simulink model "VSMr_2023b"  (R2023b)
settings: Solver=ode14x  StartTime=0  StopTime=Sim.tend  FixedStep=0.000125  RelTol=4e-4
model workspace (MAT data in the model file):
  nr_vsm : Simulink.Parameter (value not decoded)
values from neighbouring files (symbols this model uses):
  ControlSampleTime = 1/8000    (= 0.000125)    [sim3run_390.m]
  ddfmax = 60    [prm3var_390.m]
  T_seccontrol = 20    [prm3var_390.m]
  Ts = TS    [sim3run_390.m]
  TVRint = 0.85    [prm3var_390.m]
  vsm_Tdaco = 0.01    [prm3var_390.m]
symbols that are objects in the model workspace (value not decoded): nr_vsm
undefined symbols (not defined in the file or in its folder): DiscIntNeverNeededParam, General, parameterset, prm_vsm, pu_vsm, UFLS, VSM
libraries: simulink x55, FriedrichLibrary x10, simulink_extras x2, spsSampleandHoldLib x2
(part 2 of 3)

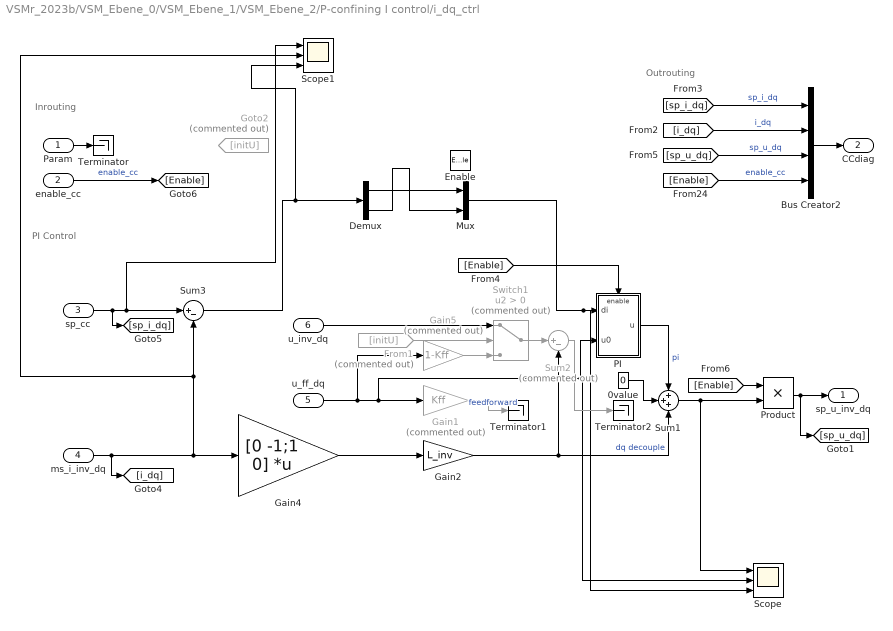
== system VSMr_2023b/VSM_Ebene_0/VSM_Ebene_1/VSM_Ebene_2/P-confining I control/i_dq_ctrl ==
  note: Inrouting
  note: Outrouting
  note: PI Control
  Param : Inport
  enable_cc : Inport  Port=2
  sp_cc : Inport  Port=3
  ms_i_inv_dq : Inport  Port=4
  u_ff_dq : Inport  Port=5
  u_inv_dq : Inport  Port=6
  Enable : EnablePort  StatesWhenEnabling=reset
  0value : Constant  Value=0
  Bus Creator2 : BusCreator  Inputs=4
  Demux : Demux  Outputs=2
  From1 : From  Commented=on  GotoTag=initU
  Gain1 : Gain  Commented=on  Gain=Kff
  Gain2 : Gain  Gain=L_inv
  Gain4 : Gain  Gain=[0 -1;1 0]  Multiplication=Matrix(K*u)
  Gain5 : Gain  Commented=on  Gain=1-Kff
  Goto2 : Goto  Commented=on  GotoTag=initU
  Mux : Mux  Inputs=2
  PI : Subsystem
  Product : Product
  Scope : Scope  NumInputPorts=3
  Scope1 : Scope  NumInputPorts=3
  Sum1 : Sum  Inputs=+++
  Sum2 : Sum  Commented=on  Inputs=|+-
  Sum3 : Sum  Inputs=|+-
  Switch1 : Switch  Commented=on  Criteria=u2 > Threshold  SaturateOnIntegerOverflow=off  InputSameDT=off
  Terminator : Terminator
  Terminator1 : Terminator
  Terminator2 : Terminator
  sp_u_inv_dq : Outport  VectorParamsAs1DForOutWhenUnconnected=off
  CCdiag : Outport  Port=2  VectorParamsAs1DForOutWhenUnconnected=off
  wires:
  Switch1/1 -> Sum2/1
  Gain4/1 -> Gain2/1
  Gain2/1 -> Sum1/3, Sum2/2  "dq decouple"
  From1/1 -> Switch1/2
  Sum1/1 -> Scope/1, Product/2
  u_inv_dq/1 -> Switch1/1
  [Enable] -> PI/Enable
  Sum3/1 -> Demux/1, Scope1/3
  sp_cc/1 -> [sp_i_dq], Scope1/1, Sum3/1
  Param/1 -> Terminator/1
  [Enable] -> Product/1
  [sp_u_dq] -> Bus Creator2/3  "sp_u_dq"
  enable_cc/1 -> [Enable]  "enable_cc"
  [Enable] -> Bus Creator2/4  "enable_cc"
  Bus Creator2/1 -> CCdiag/1
  [sp_i_dq] -> Bus Creator2/1  "sp_i_dq"
  [i_dq] -> Bus Creator2/2  "i_dq"
  u_ff_dq/1 -> PI/2(u0), Scope/2, Gain1/1, Gain5/1
  Gain5/1 -> Switch1/3
  Product/1 -> sp_u_inv_dq/1, [sp_u_dq]
  ms_i_inv_dq/1 -> [i_dq], Scope1/2, Sum3/2, Gain4/1
  Mux/1 -> Scope/3, PI/1(di)
  Demux/2 -> Mux/2
  Demux/1 -> Mux/1
  PI/1(u) -> Sum1/1  "pi"
  Gain1/1 -> Terminator1/1  "feedforward"
  Sum2/1 -> Terminator2/1
  0value/1 -> Sum1/2

== system VSMr_2023b/VSM_Ebene_0/VSM_Ebene_1/VSM_Ebene_2/VSM_Ebene_3/Angle Integrator [SI] ==
  omega : Inport
  phi0 : Inport  Port=2
  Bias : Bias  Bias=-2*pi  SaturateOnIntegerOverflow=off
  Bias1 : Bias  Bias=2*pi  SaturateOnIntegerOverflow=off
  Delay : Delay  DelayLength=1  InitialConditionSource=Input port  SampleTime=Ts
      settings: InputPortMap=u0,p4
  Delay1 : Delay  DelayLength=1  InitialConditionSource=Input port  SampleTime=Ts
      settings: InputPortMap=u0,p4
  Gain3 : Gain  Gain=Ts
  Sum : Sum  Inputs=|++
  Sum1 : Sum  Inputs=|++
  Switch : Switch  Criteria=u2 > Threshold  Threshold=pi  SaturateOnIntegerOverflow=off  InputSameDT=off
  Switch1 : Switch  Threshold=-pi  SaturateOnIntegerOverflow=off  InputSameDT=off
  phi : Outport  VectorParamsAs1DForOutWhenUnconnected=off
  phi_acc : Outport  Port=2  VectorParamsAs1DForOutWhenUnconnected=off
  wires:
  Delay1/1 -> Sum1/2, phi_acc/1
  Sum1/1 -> Delay1/1
  Gain3/1 -> Sum/1, Sum1/1
  phi0/1 -> Delay/2, Delay1/2
  omega/1 -> Gain3/1
  Bias/1 -> Switch/1
  Sum/1 -> Switch/3, Switch/2, Bias/1
  Delay/1 -> Sum/2, phi/1
  Switch/1 -> Switch1/1, Bias1/1, Switch1/2
  Bias1/1 -> Switch1/3
  Switch1/1 -> Delay/1

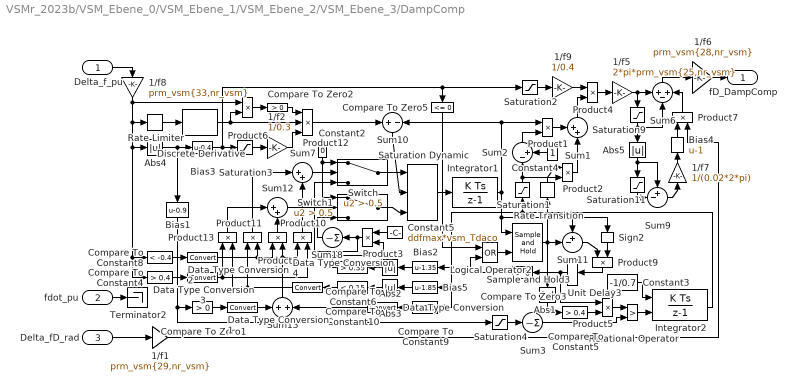
== system VSMr_2023b/VSM_Ebene_0/VSM_Ebene_1/VSM_Ebene_2/VSM_Ebene_3/DampComp ==
  Delta_f_pu : Inport
  fdot_pu : Inport  Port=2
  Delta_fD_rad : Inport  Port=3
  1/f1 : Gain  Gain=prm_vsm{29,nr_vsm}
  1/f2 : Gain  Gain=1/0.3
  1/f5 : Gain  Gain=2*pi*prm_vsm{25,nr_vsm}
  1/f6 : Gain  Gain=prm_vsm{28,nr_vsm}
  1/f7 : Gain  Gain=1/(0.02*2*pi)
  1/f8 : Gain  Gain=prm_vsm{33,nr_vsm}
  1/f9 : Gain  Gain=1/0.4
  Abs{1..5} (5 alike) : Abs  SaturateOnIntegerOverflow=off
  Bias1 : Bias  Bias=-0.9  SaturateOnIntegerOverflow=off
  Bias2 : Bias  Bias=-1.35  SaturateOnIntegerOverflow=off
  Bias3 : Bias  Bias=-0.4  SaturateOnIntegerOverflow=off
  Bias4 : Bias  Bias=-1  SaturateOnIntegerOverflow=off
  Bias5 : Bias  Bias=-1.85  SaturateOnIntegerOverflow=off
  Compare To Constant10 : simulink/Logic and Bit Operations/Compare To Constant  relop=<  const=0.15  OutDataTypeStr=boolean
  Compare To Constant4 : simulink/Logic and Bit Operations/Compare To Constant  relop=>  const=0.4  OutDataTypeStr=boolean
  Compare To Constant5 : simulink/Logic and Bit Operations/Compare To Constant  relop=>  const=0.4  OutDataTypeStr=boolean
  Compare To Constant6 : simulink/Logic and Bit Operations/Compare To Constant  relop=>  const=0.35  OutDataTypeStr=boolean
  Compare To Constant8 : simulink/Logic and Bit Operations/Compare To Constant  relop=<  const=-0.4  OutDataTypeStr=boolean
  Compare To Constant9 : simulink/Logic and Bit Operations/Compare To Constant  relop=<  const=1.5  OutDataTypeStr=boolean
  Compare To Zero1 : simulink/Logic and Bit Operations/Compare To Zero  relop=>  OutDataTypeStr=boolean
  Compare To Zero2 : simulink/Logic and Bit Operations/Compare To Zero  relop=>  OutDataTypeStr=boolean
  Compare To Zero3 : simulink/Logic and Bit Operations/Compare To Zero  relop=>  OutDataTypeStr=boolean
  Compare To Zero5 : simulink/Logic and Bit Operations/Compare To Zero  relop=<=  OutDataTypeStr=boolean
  Constant2 : Constant  Value=0
  Constant3 : Constant  Value=-1/0.7
  Constant4 : Constant
  Constant5 : Constant  Value=ddfmax*vsm_Tdaco
  Data Type Conversion{,1..4} (5 alike) : DataTypeConversion  SaturateOnIntegerOverflow=off  RndMeth=Floor
  Discrete Derivative : simulink/Discrete/Discrete Derivative  gainval=1.0  ICPrevScaledInput=0.0  OutMin=[]  OutMax=[]  OutDataType=fixdt(1, 16)  OutScaling=2^-10  DoSatur=off
  Integrator1 : DiscreteIntegrator  gainval=1/vsm_Tdaco  SampleTime=-1  LimitOutput=on  UpperSaturationLimit=4  LowerSaturationLimit=-4  ICPrevOutput=DiscIntNeverNeededParam  ICPrevScaledInput=DiscIntNeverNeededParam
  Integrator2 : DiscreteIntegrator  gainval=1  ExternalReset=level  InitialCondition=2.001  SampleTime=-1  LimitOutput=on  UpperSaturationLimit=2.001  LowerSaturationLimit=0  ICPrevOutput=DiscIntNeverNeededParam  ICPrevScaledInput=DiscIntNeverNeededParam
  Logical Operator2 : Logic  Operator=OR  AllPortsSameDT=off  OutDataTypeStr=boolean
  Product{1..11,13} (12 alike) : Product
  Product12 : Product  Inputs=3
  Rate Limiter : RateLimiter  RisingSlewLimit=4  FallingSlewLimit=-4  SampleTimeMode=inherited
  Rate Transition : RateTransition  Integrity=off  InitialCondition=-1  OutPortSampleTime=ControlSampleTime
  Relational Operator : RelationalOperator  Operator=>  OutDataTypeStr=boolean  RndMeth=Simplest  InputSameDT=off
  Sample and Hold3 : spsSampleandHoldLib/Sample and Hold  ic=0  Ts=0
  Saturation Dynamic : simulink/Discontinuities/Saturation Dynamic  OutMin=[]  OutMax=[]  OutDataTypeStr=Inherit: Same as second input  OutDataType=fixdt(1, 16)  OutScaling=2^-10  DoSatur=off
  Saturation1 : Saturate  UpperLimit=1  LowerLimit=0
  Saturation11 : Saturate  UpperLimit=0.02*2*pi  LowerLimit=0
  Saturation2 : Saturate  UpperLimit=0.4  LowerLimit=0
  Saturation3 : Saturate  UpperLimit=0.3  LowerLimit=0
  Saturation4 : Saturate  UpperLimit=0.3  LowerLimit=0.01
  Saturation9 : Saturate  UpperLimit=0.04*2*pi  LowerLimit=-0.04*2*pi
  Sign2 : Signum
  Sum1 : Sum  Inputs=++|
  Sum10 : Sum  Inputs=+|-
  Sum11 : Sum  Inputs=+-|
  Sum12 : Sum  Inputs=|++
  Sum13 : Sum  Inputs=+|+
  Sum18 : Sum  Inputs=|-|
  Sum2 : Sum  Inputs=|-+
  Sum3 : Sum  Inputs=-
  Sum6 : Sum  Inputs=+-+
  Sum7 : Sum  Inputs=|++
  Sum9 : Sum  Inputs=+-|
  Switch : Switch  Criteria=u2 > Threshold  Threshold=0.5  SaturateOnIntegerOverflow=off  InputSameDT=off
  Switch1 : Switch  Criteria=u2 > Threshold  Threshold=0.5  SaturateOnIntegerOverflow=off  InputSameDT=off
  Terminator2 : Terminator
  Unit Delay3 : UnitDelay  SampleTime=-1  HasFrameUpgradeWarning=on
  fD_DampComp : Outport
  wires:
  fdot_pu/1 -> Terminator2/1
  Delta_f_pu/1 -> 1/f8/1
  Delta_fD_rad/1 -> 1/f1/1
  Product7/1 -> Sum6/3
  Saturation9/1 -> Sum6/2, Abs5/1
  1/f7/1 -> Bias4/1
  Abs5/1 -> Sum9/1, Saturation11/1
  Saturation11/1 -> Sum9/2
  Sum9/1 -> 1/f7/1
  Bias4/1 -> Product7/1
  1/f5/1 -> Sum6/1, Saturation9/1
  1/f8/1 -> Abs4/1, Compare To Constant4/1, Compare To Constant8/1, Rate Limiter/1, Product6/1
  Sum10/1 -> Saturation Dynamic/2
  Product12/1 -> Sum10/1
  Saturation Dynamic/1 -> Integrator1/1
  Bias3/1 -> Saturation2/1, Compare To Zero5/1, Saturation3/1
  Integrator1/1 -> Product1/1, Sum10/2, Sample and Hold3/1, Sign2/1, Sum11/1
  Sum11/1 -> Product9/1
  Product5/1 -> Relational Operator/1
  Switch/1 -> Saturation Dynamic/1
  Constant2/1 -> Switch1/1, Switch/1
  Switch1/1 -> Saturation Dynamic/3
  Product3/1 -> Switch/3, Sum18/1
  Sum18/1 -> Switch1/3
  Sum6/1 -> 1/f6/1
  1/f1/1 -> Product7/2
  Compare To Zero5/1 -> Logical Operator2/1
  Product4/1 -> 1/f5/1
  Product2/1 -> Sum1/2
  Product1/1 -> Sum1/1
  Saturation1/1 -> Sum2/1, Product2/2
  Compare To Zero3/1 -> Logical Operator2/2
  Sum2/1 -> Product1/2
  Sample and Hold3/1 -> Rate Transition/1, Abs1/1, Sum11/2
  Constant5/1 -> Product3/1
  1/f6/1 -> fD_DampComp/1
  Sum1/1 -> Product4/2
  1/f9/1 -> Product4/1
  Saturation2/1 -> 1/f9/1
  1/f2/1 -> Product12/3
  Abs1/1 -> Compare To Constant5/1
  Compare To Constant5/1 -> Product5/2
  Product6/1 -> Compare To Zero2/1
  Compare To Zero2/1 -> Product12/1
  Bias2/1 -> Abs2/1
  Abs2/1 -> Compare To Constant6/1
  Compare To Constant6/1 -> Product3/2
  Sum7/1 -> Switch/2
  Compare To Constant4/1 -> Data Type Conversion3/1
  Sum12/1 -> Switch1/2
  Compare To Constant8/1 -> Data Type Conversion2/1
  Unit Delay3/1 -> Compare To Zero3/1, Product5/1
  Relational Operator/1 -> Integrator2/2
  Integrator2/1 -> Bias2/1, Bias5/1, Compare To Constant9/1, Saturation1/1
  Compare To Constant9/1 -> Data Type Conversion/1
  Bias5/1 -> Abs3/1
  Abs3/1 -> Compare To Constant10/1
  Product8/1 -> Sum12/2
  Sum13/1 -> Product8/2, Product10/1
  Abs4/1 -> Bias1/1, Bias3/1
  Product10/1 -> Sum7/2
  Product13/1 -> Sum12/1
  Compare To Constant10/1 -> Data Type Conversion4/1
  Product11/1 -> Sum7/1
  Data Type Conversion/1 -> Sum13/2
  Data Type Conversion1/1 -> Sum13/1
  Data Type Conversion2/1 -> Product11/2, Product8/1
  Data Type Conversion3/1 -> Product13/1, Product10/2
  Data Type Conversion4/1 -> Product11/1, Product13/2
  Discrete Derivative/1 -> Product12/2, Product6/2
  Rate Limiter/1 -> Discrete Derivative/1
  Sign2/1 -> Product9/2
  Saturation3/1 -> 1/f2/1
  Compare To Zero1/1 -> Data Type Conversion1/1
  Bias1/1 -> Saturation4/1, Compare To Zero1/1
  Sum3/1 -> Relational Operator/2
  Saturation4/1 -> Sum3/1
  Rate Transition/1 -> Product2/1
  Constant3/1 -> Integrator2/1
  Constant4/1 -> Sum2/2
  Product9/1 -> Unit Delay3/1
  Logical Operator2/1 -> Sample and Hold3/2

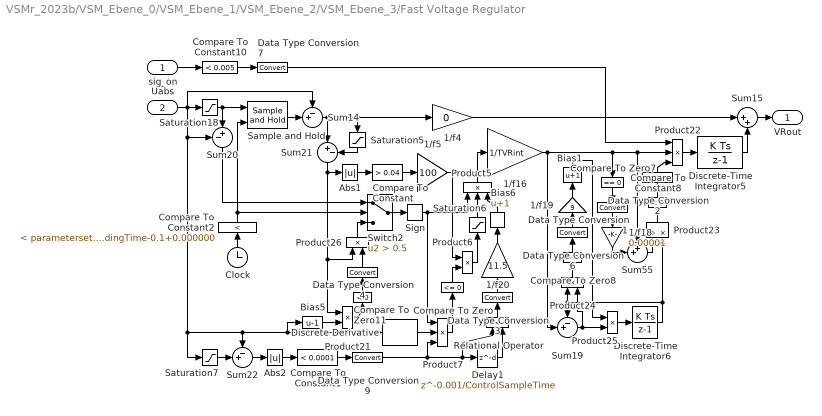
== system VSMr_2023b/VSM_Ebene_0/VSM_Ebene_1/VSM_Ebene_2/VSM_Ebene_3/Fast Voltage Regulator ==
  sig_on : Inport
  Uabs : Inport  Port=2  SampleTime=ControlSampleTime
  1/f16 : Gain  Gain=1/TVRint
  1/f18 : Gain  Gain=0.00001
  1/f19 : Gain  Gain=9
  1/f20 : Gain  Gain=11.5
  1/f4 : Gain  Gain=0
  1/f5 : Gain  Gain=100
  Abs1 : Abs  SaturateOnIntegerOverflow=off
  Abs2 : Abs  SaturateOnIntegerOverflow=off
  Bias1 : Bias  Bias=1  SaturateOnIntegerOverflow=off
  Bias5 : Bias  Bias=-1  SaturateOnIntegerOverflow=off
  Bias6 : Bias  Bias=1  SaturateOnIntegerOverflow=off
  Clock : Clock
  Compare To Constant : simulink/Logic and Bit Operations/Compare To Constant  relop=>  const=0.04  OutDataTypeStr=boolean
  Compare To Constant1 : simulink/Logic and Bit Operations/Compare To Constant  relop=<  const=0.0001  OutDataTypeStr=boolean
  Compare To Constant10 : simulink/Logic and Bit Operations/Compare To Constant  relop=<  const=0.005  OutDataTypeStr=boolean
  Compare To Constant2 : simulink/Logic and Bit Operations/Compare To Constant  relop=<  const=parameterset.Event.IslandingTime-0.1+0.000000  OutDataTypeStr=boolean
  Compare To Constant8 : simulink/Logic and Bit Operations/Compare To Constant  relop=<  const=2  OutDataTypeStr=boolean
  Compare To Zero : simulink/Logic and Bit Operations/Compare To Zero  relop=<=  OutDataTypeStr=boolean
  Compare To Zero11 : simulink/Logic and Bit Operations/Compare To Zero  relop=<  OutDataTypeStr=boolean
  Compare To Zero7 : simulink/Logic and Bit Operations/Compare To Zero  relop===  OutDataTypeStr=boolean
  Compare To Zero8 : simulink/Logic and Bit Operations/Compare To Zero  relop=>  OutDataTypeStr=boolean
  Data Type Conversion{1..4,6..7,9} (7 alike) : DataTypeConversion  SaturateOnIntegerOverflow=off  RndMeth=Floor
  Delay1 : Delay  DelayLength=0.001/ControlSampleTime  InitialCondition=0
  Discrete Derivative : simulink/Discrete/Discrete Derivative  gainval=1.0  ICPrevScaledInput=0.0  OutMin=[]  OutMax=[]  OutDataType=fixdt(1, 16)  OutScaling=2^-10  DoSatur=off
  Discrete-Time Integrator5 : DiscreteIntegrator  gainval=1  InitialCondition=0.1  SampleTime=-1  LimitOutput=on  UpperSaturationLimit=1  LowerSaturationLimit=-0.4  ICPrevOutput=DiscIntNeverNeededParam  ICPrevScaledInput=DiscIntNeverNeededParam
  Discrete-Time Integrator6 : DiscreteIntegrator  gainval=1/0.01  SampleTime=-1  ICPrevOutput=DiscIntNeverNeededParam  ICPrevScaledInput=DiscIntNeverNeededParam
  Product{6,21,24..26} (5 alike) : Product
  Product22 : Product  Inputs=3
  Product23 : Product  Inputs=/*
  Product5 : Product  Inputs=3
  Product7 : Product  Inputs=3
  Relational Operator : RelationalOperator  Operator=<  OutDataTypeStr=boolean  RndMeth=Simplest  InputSameDT=off
  Sample and Hold : spsSampleandHoldLib/Sample and Hold  ic=1  Ts=0
  Saturation18 : Saturate  UpperLimit=prm_vsm{36,nr_vsm}  LowerLimit=prm_vsm{37,nr_vsm}
  Saturation5 : Saturate  UpperLimit=0.01  LowerLimit=-0.01
  Saturation6 : Saturate  UpperLimit=10  LowerLimit=1
  Saturation7 : Saturate  UpperLimit=1.08  LowerLimit=0.9
  Sign : Signum
  Sum{14,19..20,22} (4 alike) : Sum  Inputs=-+|
  Sum15 : Sum  Inputs=|++
  Sum21 : Sum  Inputs=|+-
  Sum55 : Sum  Inputs=++|
  Switch2 : Switch  Criteria=u2 > Threshold  Threshold=0.5  SaturateOnIntegerOverflow=off  InputSameDT=off
  VRout : Outport
  wires:
  Bias5/1 -> Product21/2
  Data Type Conversion7/1 -> Product22/1
  Sign/1 -> Product5/1, Product7/1
  Bias6/1 -> Product5/3
  Compare To Constant2/1 -> Sample and Hold/2, Switch2/2
  Product24/1 -> Compare To Zero8/1
  1/f20/1 -> Bias6/1
  Product5/1 -> 1/f16/1
  Compare To Constant/1 -> 1/f5/1
  Sum14/1 -> 1/f4/1, Saturation5/1, Sum21/1
  Compare To Zero/1 -> Product6/2
  Product26/1 -> Switch2/3
  Uabs/1 -> Sum14/1, Saturation18/1, Sum20/1, Saturation7/1, Bias5/1, Discrete Derivative/1, Sum22/1
  Sum55/1 -> Product23/1
  Compare To Zero7/1 -> Data Type Conversion1/1
  Compare To Constant1/1 -> Data Type Conversion9/1
  Relational Operator/1 -> Data Type Conversion3/1
  1/f16/1 -> Product22/2, Sum55/1, Compare To Zero7/1, Sum19/2
  Compare To Constant8/1 -> Data Type Conversion2/1
  1/f4/1 -> Sum15/1
  Saturation7/1 -> Sum22/2
  1/f5/1 -> Product6/1
  Discrete-Time Integrator5/1 -> Sum15/2
  Product6/1 -> Saturation6/1
  Sample and Hold/1 -> Sum14/2
  Bias1/1 -> Product25/1
  1/f19/1 -> Bias1/1
  Switch2/1 -> Sign/1
  Product22/1 -> Discrete-Time Integrator5/1
  Sum19/1 -> Product25/2, Product24/2
  Data Type Conversion6/1 -> 1/f19/1
  Discrete-Time Integrator6/1 -> Product24/1, Sum19/1, Product23/2
  Sum22/1 -> Abs2/1
  Delay1/1 -> Relational Operator/2
  sig_on/1 -> Compare To Constant10/1
  Product25/1 -> Discrete-Time Integrator6/1
  Product23/1 -> Compare To Constant8/1
  Compare To Constant10/1 -> Data Type Conversion7/1
  Product21/1 -> Compare To Zero11/1
  Sum21/1 -> Product21/1, Product26/1, Abs1/1
  1/f18/1 -> Sum55/2
  Data Type Conversion9/1 -> Relational Operator/1, Delay1/1, Product7/3
  Discrete Derivative/1 -> Product7/2
  Saturation6/1 -> Product5/2
  Product7/1 -> Compare To Zero/1
  Abs2/1 -> Compare To Constant1/1
  Clock/1 -> Compare To Constant2/1
  Abs1/1 -> Compare To Constant/1
  Sum20/1 -> Switch2/1
  Compare To Zero8/1 -> Data Type Conversion6/1
  Saturation18/1 -> Sum20/2, Sample and Hold/1
  Compare To Zero11/1 -> Data Type Conversion4/1
  Saturation5/1 -> Sum21/2
  Sum15/1 -> VRout/1
  Data Type Conversion1/1 -> 1/f18/1
  Data Type Conversion2/1 -> Product22/3
  Data Type Conversion3/1 -> 1/f20/1
  Data Type Conversion4/1 -> Product26/2

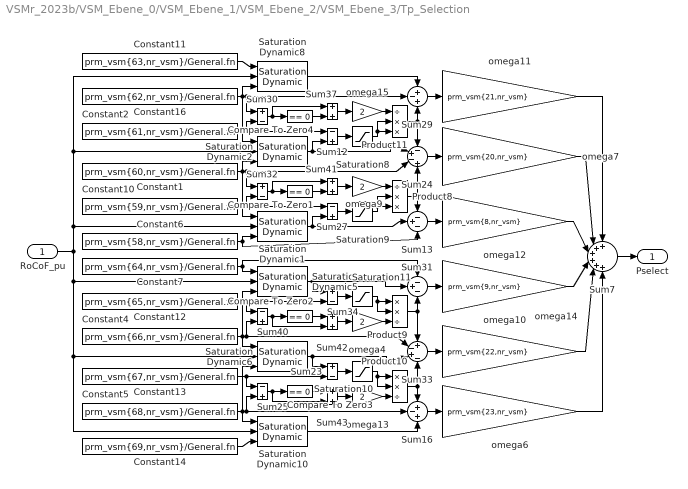
== system VSMr_2023b/VSM_Ebene_0/VSM_Ebene_1/VSM_Ebene_2/VSM_Ebene_3/Tp_Selection ==
  RoCoF_pu : Inport
  Compare To Zero{1..4} (4 alike) : simulink/Logic and Bit Operations/Compare To Zero  relop===  OutDataTypeStr=boolean
  Constant1 : Constant  Value=prm_vsm{60,nr_vsm}/General.fn
  Constant10 : Constant  Value=prm_vsm{59,nr_vsm}/General.fn
  Constant11 : Constant  Value=prm_vsm{63,nr_vsm}/General.fn
  Constant12 : Constant  Value=prm_vsm{65,nr_vsm}/General.fn
  Constant13 : Constant  Value=prm_vsm{67,nr_vsm}/General.fn
  Constant14 : Constant  Value=prm_vsm{69,nr_vsm}/General.fn
  Constant16 : Constant  Value=prm_vsm{62,nr_vsm}/General.fn
  Constant2 : Constant  Value=prm_vsm{61,nr_vsm}/General.fn
  Constant4 : Constant  Value=prm_vsm{66,nr_vsm}/General.fn
  Constant5 : Constant  Value=prm_vsm{68,nr_vsm}/General.fn
  Constant6 : Constant  Value=prm_vsm{58,nr_vsm}/General.fn
  Constant7 : Constant  Value=prm_vsm{64,nr_vsm}/General.fn
  Product10 : Product  Inputs=**/
  Product11 : Product  Inputs=/**
  Product8 : Product  Inputs=/**
  Product9 : Product  Inputs=**/
  Saturation Dynamic{1..2,5..6,8,10} (6 alike) : simulink/Discontinuities/Saturation Dynamic  OutMin=0  OutMax=[]  OutDataTypeStr=Inherit: Same as second input  OutDataType=fixdt(1, 16)  OutScaling=2^-10  DoSatur=off
  Saturation10 : Saturate  UpperLimit=0  LowerLimit=-inf
  Saturation11 : Saturate  UpperLimit=0  LowerLimit=-inf
  Saturation8 : Saturate  UpperLimit=inf  LowerLimit=0
  Saturation9 : Saturate  UpperLimit=inf  LowerLimit=0
  Sum{12,25,27,40} (4 alike) : Sum  Inputs=-+
  Sum13 : Sum  Inputs=-+-
  Sum16 : Sum  Inputs=+-+
  Sum{23,30,32,34} (4 alike) : Sum  Inputs=+-
  Sum24 : Sum  Inputs=-+-+
  Sum29 : Sum  Inputs=+-+
  Sum31 : Sum  Inputs=-+-
  Sum33 : Sum  Inputs=+-+-
  Sum{37,41..43} (4 alike) : Sum
  Sum7 : Sum  Inputs=++++++
  omega10 : Gain  Gain=prm_vsm{9,nr_vsm}
  omega11 : Gain  Gain=prm_vsm{21,nr_vsm}
  omega12 : Gain  Gain=prm_vsm{8,nr_vsm}
  omega{4,9,13,15} (4 alike) : Gain  Gain=2
  omega14 : Gain  Gain=prm_vsm{22,nr_vsm}
  omega6 : Gain  Gain=prm_vsm{23,nr_vsm}
  omega7 : Gain  Gain=prm_vsm{20,nr_vsm}
  Pselect : Outport
  wires:
  Constant6/1 -> Saturation Dynamic1/3, Sum13/3
  Constant16/1 -> Saturation Dynamic2/1, Saturation Dynamic8/3, Sum30/1, Sum29/2
  Constant5/1 -> Saturation Dynamic6/3, Sum25/2, Sum16/2, Saturation Dynamic10/1
  Constant2/1 -> Sum30/2, Sum12/1
  Saturation11/1 -> Product9/2, Product9/1
  Sum34/1 -> Saturation11/1
  RoCoF_pu/1 -> Saturation Dynamic10/2, Saturation Dynamic6/2, Saturation Dynamic5/2, Saturation Dynamic8/2, Saturation Dynamic2/2, Saturation Dynamic1/2
  Sum27/1 -> Saturation9/1
  Sum25/1 -> Sum43/2, Compare To Zero3/1
  Sum30/1 -> Sum37/1, Compare To Zero4/1
  Product8/1 -> Sum13/1, Sum24/4
  Sum33/1 -> omega14/1
  Saturation10/1 -> Product10/2, Product10/1
  Saturation Dynamic2/1 -> Sum24/2, Sum12/2
  Product9/1 -> Sum31/3, Sum33/1
  Constant12/1 -> Sum40/1, Sum34/2
  Sum29/1 -> omega11/1
  Sum13/1 -> omega12/1
  omega14/1 -> Sum7/5
  Sum16/1 -> omega6/1
  Compare To Zero2/1 -> Sum42/1
  omega13/1 -> Product10/3
  Sum32/1 -> Sum41/1, Compare To Zero1/1
  Compare To Zero1/1 -> Sum41/2
  Saturation Dynamic6/1 -> Sum33/3, Sum23/1
  Saturation9/1 -> Product8/2, Product8/3
  Sum37/1 -> omega15/1
  omega6/1 -> Sum7/6
  Sum31/1 -> omega10/1
  Sum23/1 -> Saturation10/1
  Constant7/1 -> Saturation Dynamic5/1, Sum31/1
  omega4/1 -> Product9/3
  Saturation Dynamic5/1 -> Sum34/1, Sum31/2
  Saturation Dynamic10/1 -> Sum16/3
  Constant13/1 -> Sum23/2, Sum25/1
  omega10/1 -> Sum7/4
  Saturation8/1 -> Product11/2, Product11/3
  Saturation Dynamic8/1 -> Sum29/1
  Constant14/1 -> Saturation Dynamic10/3
  Product11/1 -> Sum24/1, Sum29/3
  omega7/1 -> Sum7/2
  omega12/1 -> Sum7/3
  omega11/1 -> Sum7/1
  Sum42/1 -> omega4/1
  Constant11/1 -> Saturation Dynamic8/1
  Compare To Zero4/1 -> Sum37/2
  Sum40/1 -> Sum42/2, Compare To Zero2/1
  Saturation Dynamic1/1 -> Sum13/2, Sum27/2
  Constant10/1 -> Sum32/2, Sum27/1
  Constant1/1 -> Saturation Dynamic2/3, Sum32/1, Sum24/3, Saturation Dynamic1/1
  omega15/1 -> Product11/1
  Sum24/1 -> omega7/1
  Sum41/1 -> omega9/1
  Sum12/1 -> Saturation8/1
  omega9/1 -> Product8/1
  Sum7/1 -> Pselect/1
  Product10/1 -> Sum16/1, Sum33/4
  Sum43/1 -> omega13/1
  Compare To Zero3/1 -> Sum43/1
  Constant4/1 -> Saturation Dynamic5/3, Sum40/2, Sum33/2, Saturation Dynamic6/1

== system VSMr_2023b/VSM_Ebene_0/VSM_Ebene_1/VSM_Ebene_2/VSM_Ebene_3/UFLS ==
  f_in : Inport
  Constant10 : Constant  Value=0.275
  Constant11 : Constant  Value=0
  Constant12 : Constant  Value=0
  Constant14 : Constant  Value=0.5
  Constant2 : Constant  Value=50
  Digital Clock1 : DigitalClock  SampleTime=ControlSampleTime
  F_delay_UFLS : Subsystem
  Sum19 : Sum  Inputs=+|+
  Switch : Switch  Criteria=u2 > Threshold  Threshold=UFLS.VSM{1,nr_vsm}  SaturateOnIntegerOverflow=off  InputSameDT=off
  Switch1 : Switch  Criteria=u2 > Threshold  Threshold=UFLS.VSM{2,nr_vsm}  SaturateOnIntegerOverflow=off  InputSameDT=off
  Switch2 : Switch  Criteria=u2 > Threshold  Threshold=0.8  SaturateOnIntegerOverflow=off  InputSameDT=off
  Switch3 : Switch  Criteria=u2 > Threshold  Threshold=0.6  SaturateOnIntegerOverflow=off  InputSameDT=off
  Switch4 : Switch  Threshold=parameterset.Event.IslandingTime-0.1+9e9*(1-prm_vsm{48,nr_vsm})  SaturateOnIntegerOverflow=off  InputSameDT=off
  Unit Delay : UnitDelay  InitialCondition=1  SampleTime=-1  HasFrameUpgradeWarning=on
  signal_ufls : Outport
  wires:
  Switch3/1 -> Switch1/2
  F_delay_UFLS/1(f_delay) -> Switch2/1, Switch3/1
  Unit Delay/1 -> Switch3/2, Switch2/2
  Constant14/1 -> Switch1/1, Switch/1
  Constant10/1 -> Switch1/3, Switch/3
  Switch2/1 -> Switch/2
  Switch/1 -> Sum19/1
  Constant11/1 -> Switch2/3
  Switch1/1 -> Sum19/2
  Sum19/1 -> signal_ufls/1, Unit Delay/1
  Constant12/1 -> Switch3/3
  Digital Clock1/1 -> Switch4/2
  Constant2/1 -> Switch4/3
  Switch4/1 -> F_delay_UFLS/1(f_in)
  f_in/1 -> Switch4/1

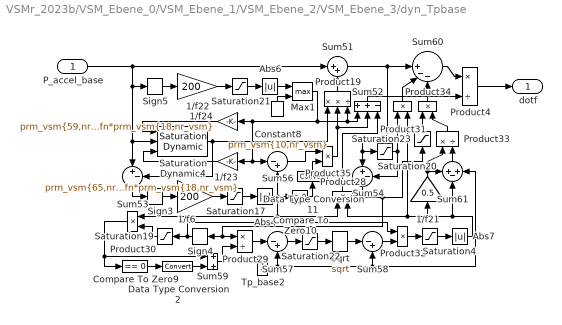
== system VSMr_2023b/VSM_Ebene_0/VSM_Ebene_1/VSM_Ebene_2/VSM_Ebene_3/dyn_Tpbase ==
  P_accel_base : Inport
  1/f21 : Gain  Gain=0.5
  1/f22 : Gain  Gain=200
  1/f23 : Gain  Gain=prm_vsm{65,nr_vsm}/General.fn*prm_vsm{18,nr_vsm}
  1/f24 : Gain  Gain=prm_vsm{59,nr_vsm}/General.fn*prm_vsm{18,nr_vsm}
  1/f6 : Gain  Gain=200
  Abs4 : Abs  SaturateOnIntegerOverflow=off
  Abs6 : Abs  SaturateOnIntegerOverflow=off
  Abs7 : Abs  SaturateOnIntegerOverflow=off
  Compare To Zero10 : simulink/Logic and Bit Operations/Compare To Zero  relop=>  OutDataTypeStr=boolean
  Compare To Zero9 : simulink/Logic and Bit Operations/Compare To Zero  relop===  OutDataTypeStr=boolean
  Constant8 : Constant  Value=prm_vsm{10,nr_vsm}
  Data Type Conversion11 : DataTypeConversion  SaturateOnIntegerOverflow=off  RndMeth=Floor
  Data Type Conversion2 : DataTypeConversion  SaturateOnIntegerOverflow=off  RndMeth=Floor
  Max1 : MinMax  Function=max  Inputs=2
  Product19 : Product  Inputs=**/
  Product{28,30..32,34..35} (6 alike) : Product
  Product29 : Product  Inputs=*/
  Product33 : Product  Inputs=*/
  Product4 : Product  Inputs=*/
  Saturation Dynamic4 : simulink/Discontinuities/Saturation Dynamic  OutMin=0  OutMax=[]  OutDataTypeStr=Inherit: Same as second input  OutDataType=fixdt(1, 16)  OutScaling=2^-10  DoSatur=off
  Saturation17 : Saturate  UpperLimit=max(prm_vsm{17,nr_vsm},prm_vsm{20,nr_vsm}*(prm_vsm{38,nr_vsm}*abs(prm_vsm{4,nr_vsm})+1-prm_vsm{38,nr_vsm}))*prm_vsm{18,nr_vsm}  LowerLimit=-(max(prm_vsm{17,nr_vsm},prm_vsm{22,nr_vsm}*(prm_vsm{38,nr_vsm}*abs(prm_vsm{5,nr_vsm})+1-prm_vsm{38,nr_vsm}))*prm_vsm{18,nr_vsm})
  Saturation19 : Saturate  UpperLimit=max(0.0001,(prm_vsm{62,nr_vsm}-prm_vsm{61,nr_vsm}))/2/General.fn  LowerLimit=min(-0.0001,(prm_vsm{68,nr_vsm}-prm_vsm{67,nr_vsm}))/2/General.fn
  Saturation20 : Saturate  UpperLimit=max(prm_vsm{17,nr_vsm},prm_vsm{20,nr_vsm}*(prm_vsm{38,nr_vsm}*abs(prm_vsm{4,nr_vsm})+1-prm_vsm{38,nr_vsm}))*prm_vsm{61,nr_vsm}/General.fn  LowerLimit=max(prm_vsm{17,nr_vsm},prm_vsm{22,nr_vsm}*(prm_vsm{38,nr_vsm}*abs(prm_vsm{5,nr_vsm})+1-prm_vsm{38,nr_vsm}))*prm_vsm{67,nr_vsm}/General.fn
  Saturation21 : Saturate  UpperLimit=prm_vsm{8,nr_vsm}*(prm_vsm{38,nr_vsm}*abs(prm_vsm{4,nr_vsm})+1-prm_vsm{38,nr_vsm})*prm_vsm{18,nr_vsm}  LowerLimit=-prm_vsm{9,nr_vsm}*(prm_vsm{38,nr_vsm}*abs(prm_vsm{5,nr_vsm})+1-prm_vsm{38,nr_vsm})*prm_vsm{18,nr_vsm}
  Saturation22 : Saturate  UpperLimit=1  LowerLimit=0
  Saturation23 : Saturate  UpperLimit=(prm_vsm{62,nr_vsm}-prm_vsm{61,nr_vsm})/General.fn/2*(1-(prm_vsm{17,nr_vsm}/max(prm_vsm{17,nr_vsm},prm_vsm{20,nr_vsm}*(prm_vsm{38,nr_vsm}*abs(prm_vsm{4,nr_vsm})+1-prm_vsm{38,nr_vsm})))^2)*max(prm_vsm{17,nr_vsm},prm_vsm{20,nr_vsm}*(prm_vsm{38,nr_vsm}*abs(prm_vsm{4,nr_vsm})+1-prm_vsm{38,nr_vsm}))  LowerLimit=(prm_vsm{68,nr_vsm}-prm_vsm{67,nr_vsm})/General.fn/2*(1-(prm_vsm{17,nr_vsm}/max(prm_vsm{17,nr_vsm},prm_vsm{22,nr_vsm}*(prm_vsm{38,nr_vsm}*abs(prm_vsm{5,nr_vsm})+1-prm_vsm{38,nr_vsm})))^2)*max(prm_vsm{17,nr_vsm},prm_vsm{22,nr_vsm}*(prm_vsm{38,nr_vsm}*abs(prm_vsm{5,nr_vsm})+1-prm_vsm{38,nr_vsm}))
  Saturation4 : Saturate  UpperLimit=min(min(sign(max(0,0.1-prm_vsm{21,nr_vsm})),sign(max(0,prm_vsm{20,nr_vsm}-prm_vsm{17,nr_vsm}))),1-prm_vsm{17,nr_vsm}/max(prm_vsm{17,nr_vsm},prm_vsm{20,nr_vsm}*(prm_vsm{38,nr_vsm}*abs(prm_vsm{4,nr_vsm})+1-prm_vsm{38,nr_vsm})))*prm_vsm{18,nr_vsm}  LowerLimit=-(min(min(sign(max(0,0.1-prm_vsm{23,nr_vsm})),sign(max(0,prm_vsm{22,nr_vsm}-prm_vsm{17,nr_vsm}))),1-prm_vsm{17,nr_vsm}/max(prm_vsm{17,nr_vsm},prm_vsm{22,nr_vsm}*(prm_vsm{38,nr_vsm}*abs(prm_vsm{5,nr_vsm})+1-prm_vsm{38,nr_vsm}))))*prm_vsm{18,nr_vsm}
  Sign3 : Signum
  Sign4 : Signum
  Sign5 : Signum
  Sqrt : Sqrt
  Sum51 : Sum  Inputs=|++
  Sum52 : Sum  Inputs=++-
  Sum53 : Sum  Inputs=|+-
  Sum54 : Sum  Inputs=|+-
  Sum56 : Sum  Inputs=|-+
  Sum57 : Sum  Inputs=|-+
  Sum58 : Sum  Inputs=|-+
  Sum59 : Sum
  Sum60 : Sum  Inputs=||+--
  Sum61 : Sum  Inputs=+-+
  Tp_base2 : Constant
  dotf : Outport
  wires:
  Saturation23/1 -> Product34/1
  Sign4/1 -> Product32/1, Saturation19/1
  Abs7/1 -> Product31/2, Product28/2, 1/f21/1, Sum61/2
  Sum52/1 -> Product4/2
  Sum54/1 -> Saturation23/1, Product29/1, Sign4/1
  Sum59/1 -> Product29/2
  Max1/1 -> 1/f24/1, Sum56/1, 1/f23/1, Product19/3, Sum52/1
  Saturation4/1 -> Abs7/1
  1/f23/1 -> Saturation Dynamic4/3
  Product28/1 -> Sum52/3
  Product19/1 -> Sum51/2
  Product34/1 -> Sum60/3
  Tp_base2/1 -> Sum61/3, Sum58/2, Sum57/2
  1/f6/1 -> Saturation17/1
  Sum61/1 -> Product33/2
  Product30/1 -> Compare To Zero9/1, Sum59/1
  Saturation19/1 -> Product30/2
  Sum60/1 -> Product4/1
  Sum58/1 -> Product32/2
  Data Type Conversion11/1 -> Product35/2
  Sign5/1 -> 1/f22/1
  Abs4/1 -> Compare To Zero10/1, Product28/1, Product30/1, Sum56/2
  Product35/1 -> Sum52/2, Product19/2
  Saturation17/1 -> Abs4/1
  Sum56/1 -> Product35/1
  Abs6/1 -> Max1/1
  Product4/1 -> dotf/1
  1/f22/1 -> Saturation21/1
  P_accel_base/1 -> Sum51/1, Sum53/1, Saturation Dynamic4/2, Sign5/1
  Saturation Dynamic4/1 -> Product19/1, Sum53/2
  Sum57/1 -> Saturation22/1
  Product31/1 -> Sum60/2
  Sum53/1 -> Sign3/1
  Sum51/1 -> Sum60/1, Saturation20/1, Sum54/1
  Saturation20/1 -> Sum54/2, Product31/1
  Compare To Zero10/1 -> Data Type Conversion11/1
  Data Type Conversion2/1 -> Sum59/2
  Saturation22/1 -> Sqrt/1
  Constant8/1 -> Max1/2
  Compare To Zero9/1 -> Data Type Conversion2/1
  Sign3/1 -> 1/f6/1
  Product32/1 -> Saturation4/1
  Sqrt/1 -> Sum58/1
  Saturation21/1 -> Abs6/1
  Product33/1 -> Product34/2
  1/f21/1 -> Product33/1, Sum61/1
  Product29/1 -> Sum57/1
  1/f24/1 -> Saturation Dynamic4/1

== system VSMr_2023b/VSM_Ebene_0/VSM_Ebene_1/VSM_Ebene_2/VSM_Ebene_3/reduced_inertia ==
  Delta_f_pu : Inport
  activate : Inport  Port=2
  1/f10 : Gain  Gain=2
  1/f11 : Gain  Gain=-10
  1/f13 : Gain  Gain=0.2
  1/f9 : Gain  Gain=prm_vsm{33,nr_vsm}*prm_vsm{50,nr_vsm}
  Abs3 : Abs  SaturateOnIntegerOverflow=off
  Bias4 : Bias  Bias=+1  SaturateOnIntegerOverflow=off
  Compare To Constant3 : simulink/Logic and Bit Operations/Compare To Constant  relop=>=  const=-0.04  OutDataTypeStr=boolean
  Compare To Constant4 : simulink/Logic and Bit Operations/Compare To Constant  relop=<  const=0.2  OutDataTypeStr=boolean
  Compare To Constant5 : simulink/Logic and Bit Operations/Compare To Constant  relop=>=  const=-0.08  OutDataTypeStr=boolean
  Compare To Constant6 : simulink/Logic and Bit Operations/Compare To Constant  relop=>  const=5.5  OutDataTypeStr=boolean
  Compare To Constant7 : simulink/Logic and Bit Operations/Compare To Constant  relop=>  const=1.2  OutDataTypeStr=boolean
  Compare To Zero12 : simulink/Logic and Bit Operations/Compare To Zero  relop=<  OutDataTypeStr=boolean
  Compare To Zero13 : simulink/Logic and Bit Operations/Compare To Zero  relop=>  OutDataTypeStr=boolean
  Data Type Conversion{1,12,14..15} (4 alike) : DataTypeConversion  SaturateOnIntegerOverflow=off  RndMeth=Floor
  Delay : Delay  DelayLength=0.1/ControlSampleTime  InitialCondition=0
  Discrete-Time Integrator3 : DiscreteIntegrator  gainval=1  ExternalReset=level  SampleTime=-1  LimitOutput=on  UpperSaturationLimit=10  LowerSaturationLimit=0  ICPrevOutput=DiscIntNeverNeededParam  ICPrevScaledInput=DiscIntNeverNeededParam
  Logical Operator1 : Logic  Operator=NAND  Inputs=3  AllPortsSameDT=off  OutDataTypeStr=boolean
  Logical Operator2 : Logic  Operator=OR  AllPortsSameDT=off  OutDataTypeStr=boolean
  Logical Operator3 : Logic  Inputs=3  AllPortsSameDT=off  OutDataTypeStr=boolean
  Math Function : Math  Operator=2^u
  Product15 : Product  Inputs=/*
  Product36 : Product
  Relational Operator1 : RelationalOperator  Operator=<  OutDataTypeStr=boolean  RndMeth=Simplest
  S-R Flip-Flop : simulink_extras/Flip Flops/S-R Flip-Flop  initial_condition=0
  Sum36 : Sum  Inputs=|+-
  Sum38 : Sum  Inputs=|++
  Sum44 : Sum  Inputs=+-|
  Terminator3 : Terminator
  Unit Delay : UnitDelay  SampleTime=-1  HasFrameUpgradeWarning=on
  Unit Delay2 : UnitDelay  SampleTime=-1  HasFrameUpgradeWarning=on
  divisor : Outport
  wires:
  1/f9/1 -> Abs3/1, 1/f13/1
  Logical Operator1/1 -> Data Type Conversion14/1
  S-R Flip-Flop/2 -> Terminator3/1
  Abs3/1 -> Sum44/1, Compare To Constant4/1, Delay/1, Sum36/1
  Delta_f_pu/1 -> Product36/1, 1/f9/1
  Compare To Zero12/1 -> Logical Operator3/3, Logical Operator1/3
  S-R Flip-Flop/1 -> Logical Operator2/2
  Discrete-Time Integrator3/1 -> Compare To Constant6/1, Math Function/1, Compare To Zero13/1
  Sum38/1 -> Discrete-Time Integrator3/1
  Compare To Constant5/1 -> Logical Operator1/1
  Delay/1 -> Sum36/2
  Compare To Constant4/1 -> Logical Operator2/1, S-R Flip-Flop/2
  Compare To Constant6/1 -> Data Type Conversion1/1
  Data Type Conversion14/1 -> 1/f11/1
  Product15/1 -> Sum38/1
  Bias4/1 -> Product15/1
  Logical Operator3/1 -> Data Type Conversion12/1
  Data Type Conversion1/1 -> Bias4/1
  Data Type Conversion15/1 -> Unit Delay/1, Relational Operator1/1
  Compare To Constant7/1 -> Logical Operator3/2, Logical Operator1/2
  activate/1 -> Product36/2
  1/f11/1 -> Sum38/2
  Unit Delay2/1 -> S-R Flip-Flop/1
  Compare To Constant3/1 -> Logical Operator3/1
  Data Type Conversion12/1 -> 1/f10/1
  Product36/1 -> Compare To Zero12/1
  Logical Operator2/1 -> Discrete-Time Integrator3/2
  Compare To Zero13/1 -> Data Type Conversion15/1
  Unit Delay/1 -> Relational Operator1/2
  Sum44/1 -> Compare To Constant7/1
  1/f13/1 -> Sum44/2
  Relational Operator1/1 -> Unit Delay2/1
  Sum36/1 -> Compare To Constant3/1, Compare To Constant5/1
  1/f10/1 -> Product15/2
  Math Function/1 -> divisor/1

== system VSMr_2023b/VSM_Ebene_0/VSM_Ebene_1/VSM_Ebene_2/VSM_Ebene_3/reverse_inertia ==
  Plfsm : Inport
  Pselect : Inport  Port=2
  Plimrise : Inport  Port=3
  Plimfall : Inport  Port=4
  1/f12 : Gain  Gain=1-prm_vsm{38,nr_vsm}
  1/f8 : Gain  Gain=-2*prm_vsm{39,nr_vsm}
  Compare To Zero5 : simulink/Logic and Bit Operations/Compare To Zero  relop=<=  OutDataTypeStr=boolean
  Compare To Zero6 : simulink/Logic and Bit Operations/Compare To Zero  relop=>  OutDataTypeStr=boolean
  Max : MinMax  Inputs=2
  Product12 : Product  Inputs=**/
  Product14 : Product
  Product18 : Product
  Product20 : Product
  Saturation14 : Saturate  UpperLimit=prm_vsm{38,nr_vsm}*prm_vsm{39,nr_vsm}*9e9  LowerLimit=0
  Saturation15 : Saturate  UpperLimit=(1-prm_vsm{38,nr_vsm})*prm_vsm{39,nr_vsm}  LowerLimit=0
  Saturation16 : Saturate  UpperLimit=inf  LowerLimit=0.00001
  Sign1 : Signum
  Sign2 : Signum
  Sum39 : Sum  Inputs=+++
  Sum46 : Sum  Inputs=++|
  lfsm_act : Outport
  signP : Outport  Port=2
  Pout : Outport  Port=3
  wires:
  Saturation14/1 -> Sum39/2
  Product18/1 -> Max/1
  Plimrise/1 -> Sum46/1
  Compare To Zero6/1 -> lfsm_act/1, Product12/1
  Pselect/1 -> Sign1/1, Product14/2
  Saturation15/1 -> Sum39/1
  Plfsm/1 -> Sign2/1, 1/f8/1
  Product14/1 -> Pout/1
  Sum39/1 -> Product14/1
  1/f12/1 -> Sum39/3
  Sum46/1 -> Product20/1
  Max/1 -> Compare To Zero6/1, Product12/2, Saturation14/1, Compare To Zero5/1
  Compare To Zero5/1 -> 1/f12/1
  Product12/1 -> Saturation15/1
  Sign1/1 -> signP/1, Product18/1
  Saturation16/1 -> Product12/3
  Product20/1 -> Max/2, Saturation16/1
  Sign2/1 -> Product20/2
  1/f8/1 -> Product18/2
  Plimfall/1 -> Sum46/2

== system VSMr_2023b/VSM_Ebene_0/VSM_Ebene_1/VSM_Ebene_2/VSM_Ebene_3/secondary control ==
  delta_fpu : Inport
  Clock : Clock
  Compare To Constant : simulink/Logic and Bit Operations/Compare To Constant  relop=>=  const=0.9  OutDataTypeStr=boolean
  Constant2 : Constant
  Discrete-Time Integrator4 : DiscreteIntegrator  gainval=1/(T_seccontrol)  SampleTime=-1  LimitOutput=on  UpperSaturationLimit=-prm_vsm{54,nr_vsm}  LowerSaturationLimit=-prm_vsm{53,nr_vsm}  ICPrevOutput=DiscIntNeverNeededParam  ICPrevScaledInput=DiscIntNeverNeededParam
  Discrete-Time Integrator5 : DiscreteIntegrator  gainval=1/(T_seccontrol/2)  SampleTime=-1  ICPrevOutput=DiscIntNeverNeededParam  ICPrevScaledInput=DiscIntNeverNeededParam
  Product5 : Product
  Product6 : Product
  Product9 : Product
  Saturation7 : Saturate  UpperLimit=-prm_vsm{54,nr_vsm}  LowerLimit=-prm_vsm{53,nr_vsm}
  Saturation8 : Saturate  UpperLimit=0.2/50  LowerLimit=0
  Sign2 : Signum
  Sum19 : Sum  Inputs=|++
  Sum9 : Sum  Inputs=-+|
  omega11 : Gain  Gain=(2.5-1)/(0.2/50)
  omega12 : Gain  Gain=prm_vsm{56,nr_vsm}*abs(prm_vsm{1,nr_vsm})
  P_sec_control : Outport
  wires:
  omega11/1 -> Sum19/2
  omega12/1 -> Sum9/2
  Sum19/1 -> Product5/2  "omega_radps"
  Discrete-Time Integrator4/1 -> Sign2/1, Product5/1
  Constant2/1 -> Sum19/1
  Product5/1 -> Saturation7/1
  Sign2/1 -> Product6/1
  Discrete-Time Integrator5/1 -> Sum9/1, Discrete-Time Integrator4/1
  Saturation8/1 -> omega11/1
  Compare To Constant/1 -> Product9/2
  Clock/1 -> Compare To Constant/1
  Product6/1 -> Saturation8/1
  Product9/1 -> Product6/2, omega12/1
  Sum9/1 -> Discrete-Time Integrator5/1
  Saturation7/1 -> P_sec_control/1
  delta_fpu/1 -> Product9/1

== system VSMr_2023b/VSM_Ebene_0/VSM_Ebene_1/VSM_Ebene_2/Virtual circuit daniel style/transient rv (HP)1 ==
  In1 : Inport
  Add : Sum  Inputs=+-
  Delay2 : Delay  DelayLength=1  SampleTime=TS
  Gain : Gain  Gain=TS/tau
  Gain1 : Gain
  Sum : Sum  Inputs=|++
  Sum2 : Sum  Inputs=|+-
  Out1 : Outport  VectorParamsAs1DForOutWhenUnconnected=off
  wires:
  Delay2/1 -> Add/2, Sum/2, Sum2/2
  Gain1/1 -> Add/1
  Sum/1 -> Delay2/1
  In1/1 -> Sum2/1, Gain1/1
  Add/1 -> Out1/1
  Gain/1 -> Sum/1
  Sum2/1 -> Gain/1

== system VSMr_2023b/VSM_Ebene_0/VSM_Ebene_1/VSM_Ebene_2/Virtual circuit daniel style/transient rv (HP)2 ==
  In1 : Inport
  Add : Sum  Inputs=+-
  Delay2 : Delay  DelayLength=1  SampleTime=TS
  Gain : Gain  Gain=TS/tau
  Gain1 : Gain
  Sum : Sum  Inputs=|++
  Sum2 : Sum  Inputs=|+-
  Out1 : Outport  VectorParamsAs1DForOutWhenUnconnected=off
  wires:
  Sum2/1 -> Gain/1
  Gain/1 -> Sum/1
  Add/1 -> Out1/1
  In1/1 -> Gain1/1, Sum2/1
  Sum/1 -> Delay2/1
  Gain1/1 -> Add/1
  Delay2/1 -> Add/2, Sum2/2, Sum/2

== system VSMr_2023b/VSM_Ebene_0/VSM_Ebene_1/VSM_Ebene_2/duty/Subsystem ==
  AlphaBeta0 : Inport
  Gain : Gain  Gain=1/2
  Saturation1 : Saturate  UpperLimit=1  LowerLimit=-1
  ab0->duty : Gain  Gain=[2 0 2; -1 sqrt(3) 2; -1 -sqrt(3) 2]  Multiplication=Matrix(K*u) (u vector)
  Duty : Outport  SampleTime=ControlSampleTime  VectorParamsAs1DForOutWhenUnconnected=off
  wires:
  Saturation1/1 -> Duty/1
  Gain/1 -> ab0->duty/1
  ab0->duty/1 -> Saturation1/1
  AlphaBeta0/1 -> Gain/1

== system VSMr_2023b/VSM_Ebene_0/VSM_Ebene_1/VSM_Ebene_2/P-confining I control/CC_switch/Enabled Subsystem ==
  i_abs : Inport
  i_pq : Inport  Port=2
  Enable : EnablePort
  i abs_pre : Outport
  i_pq_pre : Outport  Port=2
  wires:
  i_abs/1 -> i abs_pre/1
  i_pq/1 -> i_pq_pre/1

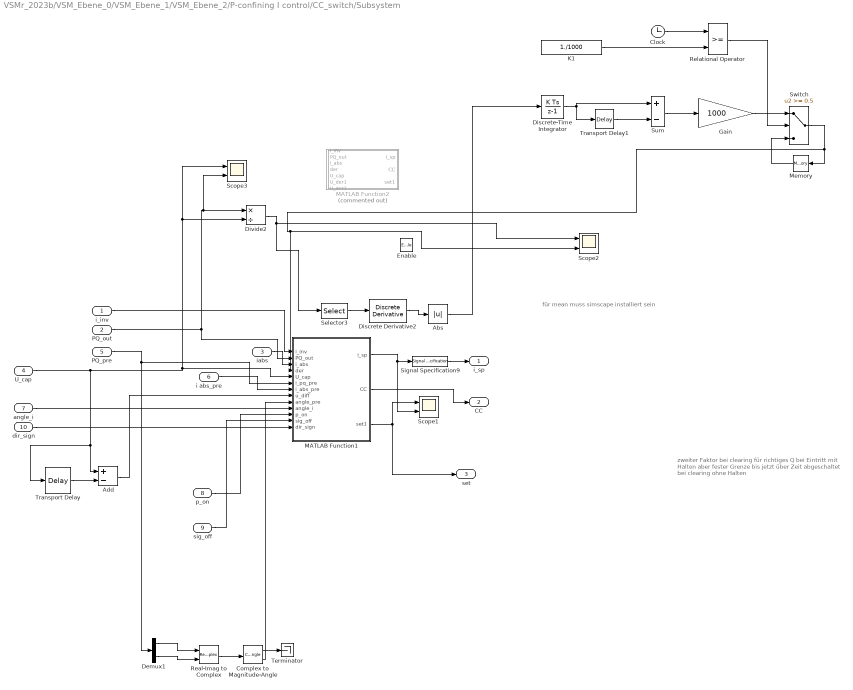
== system VSMr_2023b/VSM_Ebene_0/VSM_Ebene_1/VSM_Ebene_2/P-confining I control/CC_switch/Subsystem ==
  note: für mean muss simscape installiert sein
  note: zweiter Faktor bei clearing für richtiges Q
      |
      | bei Eintritt mit Halten aber fester Grenze
      |
      | bis jetzt über Zeit abgeschaltet bei clearing ohne Halten
  i_inv : Inport
  PQ_out : Inport  Port=2
  iabs : Inport  Port=3
  U_cap : Inport  Port=4
  PQ_pre : Inport  Port=5
  i abs_pre : Inport  Port=6
  angle_i : Inport  Port=7
  p_on : Inport  Port=8
  sig_off : Inport  Port=9
  dir_sign : Inport  Port=10
  Enable : EnablePort
  Abs : Abs  SaturateOnIntegerOverflow=off
  Add : Sum  Inputs=+-
  Clock : Clock
  Complex to Magnitude-Angle : ComplexToMagnitudeAngle
  Demux1 : Demux  Outputs=2
  Discrete Derivative2 : simulink/Discrete/Discrete Derivative  gainval=1.0  ICPrevScaledInput=0.0  OutMin=[]  OutMax=[]  OutDataType=fixdt(1, 16)  OutScaling=2^-10  DoSatur=off
  Discrete-Time Integrator : DiscreteIntegrator  SampleTime=-1  ICPrevOutput=DiscIntNeverNeededParam  ICPrevScaledInput=DiscIntNeverNeededParam
  Divide2 : Product  Inputs=*/
  Gain : Gain  Gain=1000  SaturateOnIntegerOverflow=on  OutDataTypeStr=Inherit: Same as input  ParamDataTypeStr=Inherit: Same as input
  K1 : Constant  Value=1./1000  SampleTime=Ts
  MATLAB Function1 : MATLAB Function  TreatAsAtomicUnit=on  SystemSampleTime=ControlSampleTime
  MATLAB Function2 : MATLAB Function  Commented=on  TreatAsAtomicUnit=on  SystemSampleTime=ControlSampleTime
  Memory : Memory
  Real-Imag to Complex : RealImagToComplex
  Relational Operator : RelationalOperator  OutDataTypeStr=boolean  ZeroCross=off  SampleTime=Ts  InputSameDT=off
  Scope1 : Scope  NumInputPorts=2
  Scope2 : Scope  NumInputPorts=2
  Scope3 : Scope  NumInputPorts=2
  Selector3 : Selector  InputPortWidth=2  IndexOptions=Index vector (dialog)  Indices=2  OutputSizes=1
  Signal Specification9 : SignalSpecification  Dimensions=[1 2]
  Sum : Sum  Inputs=+-  InputSameDT=on  SaturateOnIntegerOverflow=on  OutDataTypeStr=Inherit: Same as first input
  Switch : Switch  Threshold=0.5  SaturateOnIntegerOverflow=off
  Terminator : Terminator
  Transport Delay : TransportDelay  DelayTime=0.002
  Transport Delay1 : TransportDelay  DelayTime=1./1000  BufferSize=2048*4  PadeOrder=2
  i_sp : Outport
  CC : Outport  Port=2
  set : Outport  Port=3
  wires:
  PQ_out/1 -> MATLAB Function1/2(PQ_out), Scope3/2, Divide2/1
  iabs/1 -> MATLAB Function1/3(i_abs)
  U_cap/1 -> Scope3/1, Divide2/2, MATLAB Function1/5(U_cap), Add/1, Transport Delay/1
  MATLAB Function1/1(i_sp) -> Scope1/2, Signal Specification9/1
  MATLAB Function1/2(CC) -> CC/1
  i abs_pre/1 -> MATLAB Function1/7(i_abs_pre)
  Transport Delay/1 -> Add/2
  Add/1 -> MATLAB Function1/8(u_diff)
  i_inv/1 -> MATLAB Function1/1(i_inv)
  Discrete Derivative2/1 -> Abs/1
  MATLAB Function1/3(set1) -> Scope1/1, set/1
  Divide2/1 -> Selector3/1, Scope2/1
  Selector3/1 -> Discrete Derivative2/1
  Demux1/1 -> Real-Imag to Complex/1
  PQ_pre/1 -> Demux1/1, MATLAB Function1/6(i_pq_pre)
  Complex to Magnitude-Angle/2 -> MATLAB Function1/9(angle_pre)
  Demux1/2 -> Real-Imag to Complex/2
  Real-Imag to Complex/1 -> Complex to Magnitude-Angle/1
  angle_i/1 -> MATLAB Function1/10(angle_i)
  Signal Specification9/1 -> i_sp/1
  Relational Operator/1 -> Switch/2
  Memory/1 -> Switch/3
  Discrete-Time Integrator/1 -> Sum/1, Transport Delay1/1
  Sum/1 -> Gain/1
  Gain/1 -> Switch/1
  Clock/1 -> Relational Operator/1
  K1/1 -> Relational Operator/2
  Transport Delay1/1 -> Sum/2
  Abs/1 -> Discrete-Time Integrator/1
  Switch/1 -> MATLAB Function1/4(der), Scope2/2, Memory/1
  p_on/1 -> MATLAB Function1/11(p_on)
  sig_off/1 -> MATLAB Function1/12(sig_off)
  dir_sign/1 -> MATLAB Function1/13(dir_sign)
  Complex to Magnitude-Angle/1 -> Terminator/1

== system VSMr_2023b/VSM_Ebene_0/VSM_Ebene_1/VSM_Ebene_2/P-confining I control/i_dq_ctrl/PI ==
  di : Inport
  u0 : Inport  Port=2
  Enable : EnablePort  StatesWhenEnabling=reset
  Gain4 : Gain  Gain=Ki
  Gain5 : Gain  Gain=Kp
  Integrator (inertia) : DiscreteIntegrator  gainval=1  InitialConditionSource=external  InitialCondition=1  SampleTime=ControlSampleTime  ICPrevOutput=DiscIntNeverNeededParam  ICPrevScaledInput=DiscIntNeverNeededParam
  Sum2 : Sum  Inputs=++|
  u : Outport  VectorParamsAs1DForOutWhenUnconnected=off
  wires:
  u0/1 -> Integrator (inertia)/2
  Sum2/1 -> u/1
  di/1 -> Gain4/1, Gain5/1
  Integrator (inertia)/1 -> Sum2/2
  Gain4/1 -> Integrator (inertia)/1
  Gain5/1 -> Sum2/1

== system VSMr_2023b/VSM_Ebene_0/VSM_Ebene_1/VSM_Ebene_2/VSM_Ebene_3/UFLS/F_delay_UFLS ==
  f_in : Inport
  Delay : Delay  DelayLength=0.08/ControlSampleTime
  Delay1 : Delay  DelayLength=0.02/ControlSampleTime  InitialCondition=General.fn
  Delay2 : Delay  DelayLength=0.04/ControlSampleTime  InitialCondition=General.fn
  Delay3 : Delay  DelayLength=0.06/ControlSampleTime  InitialCondition=General.fn
  Delay4 : Delay  DelayLength=0.07/ControlSampleTime  InitialCondition=General.fn
  MinMax : MinMax  Function=max  Inputs=5
  f_delay : Outport
  wires:
  MinMax/1 -> Delay4/1
  f_in/1 -> Delay/1, Delay3/1, Delay2/1, Delay1/1, MinMax/1
  Delay2/1 -> MinMax/3
  Delay1/1 -> MinMax/2
  Delay3/1 -> MinMax/4
  Delay/1 -> MinMax/5
  Delay4/1 -> f_delay/1  "f_ufls"
